simulink model "ADAC_AEBS_Test_B5_cs"  (R2014b)
settings: Solver=ode5  SolverMode=SingleTasking  StartTime=0.0  StopTime=inf  FixedStep=1/100  RelTol=1e-3
PreLoadFcn:
  | mbxruntime.callbacks.PreLoadFcn(bdroot);
  | check_NUTS_defined;
  | 
  | assignin('base',['model_closed_' bdroot],false);addpath('../includes_AEBS');
PostLoadFcn:
  | mbxruntime.callbacks.PostLoadFcn(bdroot);
InitFcn:
  | mbxruntime.callbacks.InitFcn(bdroot);
StartFcn:
  | mbxruntime.callbacks.StartFcn(bdroot);
StopFcn:
  | mbxruntime.callbacks.StopFcn(bdroot);
model workspace: external: MAT-File .\ADAC_AEBS_Test_B5_cs_hws.mat (data not in the file)
undefined symbols (not defined in the file or in its folder): OrientationPitch, OrientationRoll, PositionX, PositionY, PositionZ, warningInitialVelocity, x0
undefined symbols (not defined in the file): ADAC_AEBS_Test_B5_cs_1f353852a1e4a3c9, ADAC_AEBS_Test_B5_cs_31880a8290cb7cd0, ADAC_AEBS_Test_B5_cs_5496c81c4b1e331d, ADAC_AEBS_Test_B5_cs_a5262f062dfd1c06, ADAC_AEBS_Test_B5_cs_abe98bde40d8f1df, ADAC_AEBS_Test_B5_cs_ADAC_target_1_Path_pathUniqueID, ADAC_AEBS_Test_B5_cs_Audi_A8_1_Dynamics_Simple_initialPitch, ADAC_AEBS_Test_B5_cs_Audi_A8_1_Dynamics_Simple_initialRoll, ADAC_AEBS_Test_B5_cs_Audi_A8_1_Dynamics_Simple_initialX, ADAC_AEBS_Test_B5_cs_Audi_A8_1_Dynamics_Simple_initialY, ADAC_AEBS_Test_B5_cs_Audi_A8_1_Dynamics_Simple_initialYaw, ADAC_AEBS_Test_B5_cs_Audi_A8_1_Dynamics_Simple_initialZ, ADAC_AEBS_Test_B5_cs_Sphere_1_Dynamics_Empty_STATE_Sphere_1_x0, ADAC_AEBS_Test_B5_cs_Sphere_1_Dynamics_Empty_STATE_Sphere_1_y0, ADAC_AEBS_Test_B5_cs_Sphere_1_Dynamics_Empty_STATE_Sphere_1_z0, SteeringColumn, SteeringWheel, WheelL0, WheelL1, WheelR0, WheelR1
libraries: simulink x20, simulink_extras x12, PreScanSimulinkLibrary x5, PreScanUsefulBlocks x2
(part 4 of 6)

== system ADAC_AEBS_Test_B5_cs/Sphere_1/Dynamics_Empty ==
  note: For state mode 'Dynamic' positions
      | are not taken into account, as they
      | are computed by integrating velocity.
      | Click annotation for Help.
  " " : Constant  Value=0
  Add : Sum
  Add1 : Sum
  Bus Selector : BusSelector  OutputSignals=PositionX,PositionY
  Bus Assignment : BusAssignment  AssignedSignals=PositionX,PositionY,PositionZ,OrientationRoll,OrientationPitch
  MuxState : Subsystem  Tag=mux/State  Commented=on  mask(Empty Dynamics State Block){positioningmode=on, TimeStep=1/100}
      mask prompts: positioningmode "Positioning Mode"; TimeStep "Auto Assigned: Time Step [s]"
      mask help:
      | Build the state of an actor based on user input.
      | The user can either use positioning mode or dynamics mode.
      | - When using positioning mode the position and orientation of the actor are set directly based on the input. Expected input is relative to the initial position and orientation of the actor. It's also possible to specify the velocity of the actor, though this input isn't used, only passed on.
      | - When using dynamics mode the position input is ignored. Expected input is velocity and orientation. The velocity is relative the current orientation of the actor, while orientation is relative to its initial orientation. The position of the actor is calculated based on the velocity and orientation given.
      settings: DeleteFcn=PreScanBlockDeleteFcn;
  OffsetX : Constant  Value=0
  OffsetY : Constant  Value=0
  STATE_Sphere_1 : Subsystem  Tag=mux/StatePort  Priority=0  Commented=on  LoadFcn=load PrescanStateActuatorData  mask(PreScan Sink Block: State){x0=ADAC_AEBS_Test_B5_cs_Sphere_1_Dynamics_Empty_STATE_Sphere_1_x0, y0=ADAC_AEBS_Test_B5_cs_Sphere_1_Dynamics_Empty_STATE_Sphere_1_y0, z0=ADAC_AEBS_Test_B5_cs_Sphere_1_Dynamics_Empty_STATE_Sphere_1_z0, Roll0=ADAC_AEBS_Test_B5_cs_1f353852a1e4a3c9, Pitch0=ADAC_AEBS_Test_B5_cs_5496c81c4b1e331d, Yaw0=ADAC_AEBS_Test_B5_cs_31880a8290cb7cd0, TimeStep=1/100}
      mask prompts: x0 "Ini x-position VEHICLE wrt GLOBAL axis system [m]"; y0 "Ini y-position VEHICLE wrt GLOBAL axis system [m]"; z0 "Ini z-position VEHICLE wrt GLOBAL axis system [m]"; Roll0 "Ini roll-angle BODY wrt VEHICLE axis system [deg]"; Pitch0 "Ini pitch-angle BODY wrt VEHICLE axis system [deg]"; Yaw0 "Ini yaw-angle VEHICLE wrt GLOBAL axis system [deg]"; TimeStep "Auto-Assigned: Upload Period [s]"
      mask help:
      | The Actor State contains a vector signal of size (9x1), containing the following signals:
      |
      | -  Position                  (x,y,z)                                     [m]
      | -  Velocity                  (vx,vy,vz)                               [m/s]
      | -  Angles                    (Roll, Pitch, Yaw)                   [rad]
      |
      | The Actor state is defined in the global axis system.
      | The state is superponed on the Initial position defined in the GUI.
      |
      | For more information, please click Help.
      settings: DeleteFcn=PreScanBlockDeleteFcn;
      mask Help: eval('openHelp(222)')
      mask Display: image(imread('State.png'))
  State : Outport  Tag=outport/StateOutport  SampleTime=1/100
  wires:
  " "/1 -> Bus Assignment/4, Bus Assignment/5, Bus Assignment/6
  [view] -> Bus Assignment/1, Bus Selector/1
  Bus Selector/1 -> Add/1
  Add/1 -> Bus Assignment/2
  OffsetX/1 -> Add/2
  Bus Selector/2 -> Add1/1
  Add1/1 -> Bus Assignment/3
  OffsetY/1 -> Add1/2
  Bus Assignment/1 -> State/1
  MuxState/1(state) -> STATE_Sphere_1/1(State)

== system ADAC_AEBS_Test_B5_cs/Sphere_1/SELF_Demux ==
  SELF : Inport  OutDataTypeStr=Bus: PRESCAN_SELFSENSORDATA
  Bus Selector : BusSelector  OutputSignals=PositionX,PositionY,PositionZ,OrientationRoll,OrientationPitch,OrientationYaw,Velocity,Yaw_rate,Lat,Long,Alt
  Demux2 : Demux  Outputs=3
  Gain : Gain  Gain=180/pi
  Gain1 : Gain  Gain=180/pi
  Vector Concatenate1 : Concatenate  NumInputs=3
  compas converter : Subsystem
  x [m] : Outport
  y [m] : Outport  Port=2
  z [m] : Outport  Port=3
  rotx [deg] : Outport  Port=4
  roty [deg] : Outport  Port=5
  rotz [deg] : Outport  Port=6
  GPS lat [deg] : Outport  Port=7
  GPS long [deg] : Outport  Port=8
  GPS alt [m] : Outport  Port=9
  velocity [m/s] : Outport  Port=10
  heading [deg] : Outport  Port=11
  yaw rate [deg/s] : Outport  Port=12
  wires:
  Bus Selector/11 -> GPS alt [m]/1  "<Alt>"
  Bus Selector/10 -> GPS long [deg]/1  "<Long>"
  Bus Selector/9 -> GPS lat [deg]/1  "<Lat>"
  Bus Selector/8 -> Gain1/1  "<Yaw_rate>"
  Bus Selector/7 -> velocity [m/s]/1  "<Velocity>"
  Bus Selector/6 -> compas converter/1(rotz [rad]), Vector Concatenate1/3  "<OrientationYaw>"
  Bus Selector/5 -> Vector Concatenate1/2  "<OrientationPitch>"
  Bus Selector/4 -> Vector Concatenate1/1  "<OrientationRoll>"
  Vector Concatenate1/1 -> Gain/1
  Bus Selector/3 -> z [m]/1  "<PositionZ>"
  Bus Selector/2 -> y [m]/1  "<PositionY>"
  Bus Selector/1 -> x [m]/1  "<PositionX>"
  SELF/1 -> Bus Selector/1
  Gain/1 -> Demux2/1
  Demux2/1 -> rotx [deg]/1
  Demux2/2 -> roty [deg]/1
  Demux2/3 -> rotz [deg]/1
  compas converter/1(heading [deg]) -> heading [deg]/1
  Gain1/1 -> yaw rate [deg/s]/1

== system ADAC_AEBS_Test_B5_cs/SteeringColumn_pivot_Audi_A8_1/Actuator ==
  Joint : Inport
  Bus Selector : BusSelector  OutputSignals=POSITION,ORIENTATION
  visu_Rotate : Subsystem  mask(RPYActuator){UniqueID=UniqueID, Object3DID=Rotate_ObjectID3D, TimeStep=TimeStep}
      mask prompts: UniqueID "Auto-Assigned: Unique ID"; Object3DID "Auto-Assigned: Child 3D Object ID"; TimeStep "Auto-Assigned: Upload Period [s]"
      mask help: Applies angles update to selected child object
      mask Help:
      | Applies position update to selected child object
      | 
      | - UniqueID (double)   : Unique ID of the parent actor
      | - Object3DID (string) : Name of the child 3D object
      mask Display: port_label('input', 1, ['visu_Rotate_' Object3DID])
  visu_Translate : Subsystem  mask(PositionActuator){UniqueID=UniqueID, Object3DID=Translate_ObjectID3D, TimeStep=TimeStep}
      mask prompts: UniqueID "Auto-Assigned: Unique ID"; Object3DID "Auto-Assigned: Child 3D Object ID"; TimeStep "Auto-Assigned: Upload Period [s]"
      mask help: Applies position update to selected child object
      mask Help:
      | Applies position update to selected child object
      | 
      | - UniqueID (double)   : Unique ID of the parent actor
      | - Object3DID (string) : Name of the child 3D object
      mask Display: port_label('input', 1, ['visu_Translate_' Object3DID])
  wires:
  Bus Selector/2 -> visu_Rotate/1(In1)  "<ORIENTATION>"
  Bus Selector/1 -> visu_Translate/1(In1)  "<POSITION>"
  Joint/1 -> Bus Selector/1

== system ADAC_AEBS_Test_B5_cs/SteeringWheel_pivot_Audi_A8_1/Actuator ==
  Joint : Inport
  Bus Selector : BusSelector  OutputSignals=POSITION,ORIENTATION
  visu_Rotate : Subsystem  mask(RPYActuator){UniqueID=UniqueID, Object3DID=Rotate_ObjectID3D, TimeStep=TimeStep}
      mask prompts: UniqueID "Auto-Assigned: Unique ID"; Object3DID "Auto-Assigned: Child 3D Object ID"; TimeStep "Auto-Assigned: Upload Period [s]"
      mask help: Applies angles update to selected child object
      mask Help:
      | Applies position update to selected child object
      | 
      | - UniqueID (double)   : Unique ID of the parent actor
      | - Object3DID (string) : Name of the child 3D object
      mask Display: port_label('input', 1, ['visu_Rotate_' Object3DID])
  visu_Translate : Subsystem  mask(PositionActuator){UniqueID=UniqueID, Object3DID=Translate_ObjectID3D, TimeStep=TimeStep}
      mask prompts: UniqueID "Auto-Assigned: Unique ID"; Object3DID "Auto-Assigned: Child 3D Object ID"; TimeStep "Auto-Assigned: Upload Period [s]"
      mask help: Applies position update to selected child object
      mask Help:
      | Applies position update to selected child object
      | 
      | - UniqueID (double)   : Unique ID of the parent actor
      | - Object3DID (string) : Name of the child 3D object
      mask Display: port_label('input', 1, ['visu_Translate_' Object3DID])
  wires:
  Bus Selector/2 -> visu_Rotate/1(In1)  "<ORIENTATION>"
  Bus Selector/1 -> visu_Translate/1(In1)  "<POSITION>"
  Joint/1 -> Bus Selector/1

== system ADAC_AEBS_Test_B5_cs/WheelL0_Audi_A8_1/Actuator ==
  Joint : Inport
  Bus Selector : BusSelector  OutputSignals=POSITION,ORIENTATION
  visu_Rotate : Subsystem  mask(RPYActuator){UniqueID=UniqueID, Object3DID=Rotate_ObjectID3D, TimeStep=TimeStep}
      mask prompts: UniqueID "Auto-Assigned: Unique ID"; Object3DID "Auto-Assigned: Child 3D Object ID"; TimeStep "Auto-Assigned: Upload Period [s]"
      mask help: Applies angles update to selected child object
      mask Help:
      | Applies position update to selected child object
      | 
      | - UniqueID (double)   : Unique ID of the parent actor
      | - Object3DID (string) : Name of the child 3D object
      mask Display: port_label('input', 1, ['visu_Rotate_' Object3DID])
  visu_Translate : Subsystem  mask(PositionActuator){UniqueID=UniqueID, Object3DID=Translate_ObjectID3D, TimeStep=TimeStep}
      mask prompts: UniqueID "Auto-Assigned: Unique ID"; Object3DID "Auto-Assigned: Child 3D Object ID"; TimeStep "Auto-Assigned: Upload Period [s]"
      mask help: Applies position update to selected child object
      mask Help:
      | Applies position update to selected child object
      | 
      | - UniqueID (double)   : Unique ID of the parent actor
      | - Object3DID (string) : Name of the child 3D object
      mask Display: port_label('input', 1, ['visu_Translate_' Object3DID])
  wires:
  Bus Selector/2 -> visu_Rotate/1(In1)  "<ORIENTATION>"
  Bus Selector/1 -> visu_Translate/1(In1)  "<POSITION>"
  Joint/1 -> Bus Selector/1

== system ADAC_AEBS_Test_B5_cs/WheelL1_Audi_A8_1/Actuator ==
  Joint : Inport
  Bus Selector : BusSelector  OutputSignals=POSITION,ORIENTATION
  visu_Rotate : Subsystem  mask(RPYActuator){UniqueID=UniqueID, Object3DID=Rotate_ObjectID3D, TimeStep=TimeStep}
      mask prompts: UniqueID "Auto-Assigned: Unique ID"; Object3DID "Auto-Assigned: Child 3D Object ID"; TimeStep "Auto-Assigned: Upload Period [s]"
      mask help: Applies angles update to selected child object
      mask Help:
      | Applies position update to selected child object
      | 
      | - UniqueID (double)   : Unique ID of the parent actor
      | - Object3DID (string) : Name of the child 3D object
      mask Display: port_label('input', 1, ['visu_Rotate_' Object3DID])
  visu_Translate : Subsystem  mask(PositionActuator){UniqueID=UniqueID, Object3DID=Translate_ObjectID3D, TimeStep=TimeStep}
      mask prompts: UniqueID "Auto-Assigned: Unique ID"; Object3DID "Auto-Assigned: Child 3D Object ID"; TimeStep "Auto-Assigned: Upload Period [s]"
      mask help: Applies position update to selected child object
      mask Help:
      | Applies position update to selected child object
      | 
      | - UniqueID (double)   : Unique ID of the parent actor
      | - Object3DID (string) : Name of the child 3D object
      mask Display: port_label('input', 1, ['visu_Translate_' Object3DID])
  wires:
  Bus Selector/2 -> visu_Rotate/1(In1)  "<ORIENTATION>"
  Bus Selector/1 -> visu_Translate/1(In1)  "<POSITION>"
  Joint/1 -> Bus Selector/1

== system ADAC_AEBS_Test_B5_cs/WheelR0_Audi_A8_1/Actuator ==
  Joint : Inport
  Bus Selector : BusSelector  OutputSignals=POSITION,ORIENTATION
  visu_Rotate : Subsystem  mask(RPYActuator){UniqueID=UniqueID, Object3DID=Rotate_ObjectID3D, TimeStep=TimeStep}
      mask prompts: UniqueID "Auto-Assigned: Unique ID"; Object3DID "Auto-Assigned: Child 3D Object ID"; TimeStep "Auto-Assigned: Upload Period [s]"
      mask help: Applies angles update to selected child object
      mask Help:
      | Applies position update to selected child object
      | 
      | - UniqueID (double)   : Unique ID of the parent actor
      | - Object3DID (string) : Name of the child 3D object
      mask Display: port_label('input', 1, ['visu_Rotate_' Object3DID])
  visu_Translate : Subsystem  mask(PositionActuator){UniqueID=UniqueID, Object3DID=Translate_ObjectID3D, TimeStep=TimeStep}
      mask prompts: UniqueID "Auto-Assigned: Unique ID"; Object3DID "Auto-Assigned: Child 3D Object ID"; TimeStep "Auto-Assigned: Upload Period [s]"
      mask help: Applies position update to selected child object
      mask Help:
      | Applies position update to selected child object
      | 
      | - UniqueID (double)   : Unique ID of the parent actor
      | - Object3DID (string) : Name of the child 3D object
      mask Display: port_label('input', 1, ['visu_Translate_' Object3DID])
  wires:
  Bus Selector/2 -> visu_Rotate/1(In1)  "<ORIENTATION>"
  Bus Selector/1 -> visu_Translate/1(In1)  "<POSITION>"
  Joint/1 -> Bus Selector/1

== system ADAC_AEBS_Test_B5_cs/WheelR1_Audi_A8_1/Actuator ==
  Joint : Inport
  Bus Selector : BusSelector  OutputSignals=POSITION,ORIENTATION
  visu_Rotate : Subsystem  mask(RPYActuator){UniqueID=UniqueID, Object3DID=Rotate_ObjectID3D, TimeStep=TimeStep}
      mask prompts: UniqueID "Auto-Assigned: Unique ID"; Object3DID "Auto-Assigned: Child 3D Object ID"; TimeStep "Auto-Assigned: Upload Period [s]"
      mask help: Applies angles update to selected child object
      mask Help:
      | Applies position update to selected child object
      | 
      | - UniqueID (double)   : Unique ID of the parent actor
      | - Object3DID (string) : Name of the child 3D object
      mask Display: port_label('input', 1, ['visu_Rotate_' Object3DID])
  visu_Translate : Subsystem  mask(PositionActuator){UniqueID=UniqueID, Object3DID=Translate_ObjectID3D, TimeStep=TimeStep}
      mask prompts: UniqueID "Auto-Assigned: Unique ID"; Object3DID "Auto-Assigned: Child 3D Object ID"; TimeStep "Auto-Assigned: Upload Period [s]"
      mask help: Applies position update to selected child object
      mask Help:
      | Applies position update to selected child object
      | 
      | - UniqueID (double)   : Unique ID of the parent actor
      | - Object3DID (string) : Name of the child 3D object
      mask Display: port_label('input', 1, ['visu_Translate_' Object3DID])
  wires:
  Bus Selector/2 -> visu_Rotate/1(In1)  "<ORIENTATION>"
  Bus Selector/1 -> visu_Translate/1(In1)  "<POSITION>"
  Joint/1 -> Bus Selector/1

== system ADAC_AEBS_Test_B5_cs/ADAC_target_1/SELF_Demux/compas converter ==
  rotz [rad] : Inport
  cart2compas : Subsystem
  rad2deg : Gain  Gain=180/pi
  heading [deg] : Outport
  wires:
  rad2deg/1 -> cart2compas/1(Angle [deg])
  rotz [rad]/1 -> rad2deg/1
  cart2compas/1(heading [deg]) -> heading [deg]/1

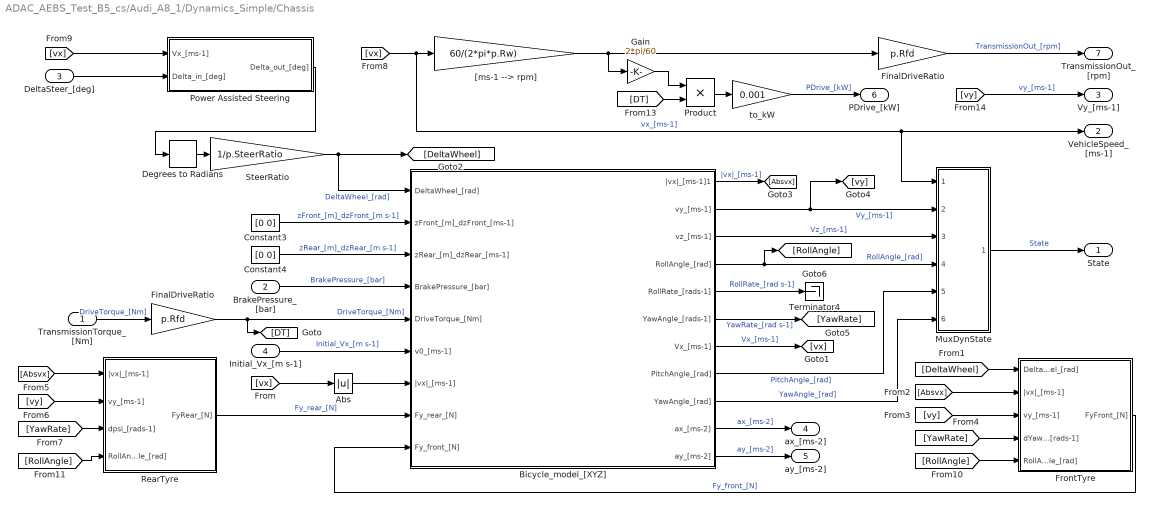
== system ADAC_AEBS_Test_B5_cs/Audi_A8_1/Dynamics_Simple/Chassis ==
  TransmissionTorque_[Nm] : Inport
  BrakePressure_[bar] : Inport  Port=2
  DeltaSteer_[deg] : Inport  Port=3
  Initial_Vx_[m s-1] : Inport  Port=4
  Abs : Abs
  Bicycle_model_[XYZ] : Subsystem
      mask Display: image(imread('Bicycle_model.png'));
  Constant3 : Constant  Value=[0 0]
  Constant4 : Constant  Value=[0 0]
  Degrees to Radians : simulink_extras/Transformations/Degrees to Radians
  FinalDriveRatio : Gain  Gain=p.Rfd  SaturateOnIntegerOverflow=on  OutDataTypeStr=Inherit: Same as input  ParamDataTypeStr=Inherit: Same as input
  "FinalDriveRatio " : Gain  Gain=p.Rfd  SaturateOnIntegerOverflow=on  OutDataTypeStr=Inherit: Same as input  ParamDataTypeStr=Inherit: Same as input
  FrontTyre : Subsystem
      mask Display: image(imread('Tyre.png'));
  Gain : Gain  Gain=2*pi/60
  MuxDynState : Subsystem
  Power Assisted Steering : Subsystem
  Product : Product  RndMeth=Zero
  RearTyre : Subsystem
      mask Display: image(imread('Tyre.png'));
  SteerRatio : Gain  Gain=1/p.SteerRatio
  Terminator4 : Terminator
  "[ms-1 --> rpm]" : Gain  Gain=60/(2*pi*p.Rw)  SaturateOnIntegerOverflow=on  OutDataTypeStr=Inherit: Same as input  ParamDataTypeStr=Inherit: Same as input
  to_kW : Gain  Gain=0.001
  State : Outport
  VehicleSpeed_[ms-1] : Outport  Port=2
  Vy_[ms-1] : Outport  Port=3
  ax_[ms-2] : Outport  Port=4
  ay_[ms-2] : Outport  Port=5
  PDrive_[kW] : Outport  Port=6
  TransmissionOut_[rpm] : Outport  Port=7
  wires:
  [vy] -> Vy_[ms-1]/1  "vy_[ms-1]"
  to_kW/1 -> PDrive_[kW]/1  "PDrive_[kW]"
  Gain/1 -> Product/1
  Bicycle_model_[XYZ]/10(ax_[ms-2]) -> ax_[ms-2]/1  "ax_[ms-2]"
  Product/1 -> to_kW/1
  [DT] -> Product/2
  Bicycle_model_[XYZ]/11(ay_[ms-2]) -> ay_[ms-2]/1  "ay_[ms-2]"
  Abs/1 -> Bicycle_model_[XYZ]/7(|vx|_[ms-1])
  Degrees to Radians/1 -> SteerRatio/1
  [vx] -> Abs/1
  SteerRatio/1 -> [DeltaWheel], Bicycle_model_[XYZ]/1(DeltaWheel_[rad])  "DeltaWheel_[rad]"
  TransmissionTorque_[Nm]/1 -> "FinalDriveRatio "/1  "DriveTorque_[Nm]"
  RearTyre/1(FyRear_[N]) -> Bicycle_model_[XYZ]/8(Fy_rear_[N])  "Fy_rear_[N]"
  FrontTyre/1(FyFront_[N]) -> Bicycle_model_[XYZ]/9(Fy_front_[N])  "Fy_front_[N]"
  Bicycle_model_[XYZ]/1(|vx|_[ms-1]1) -> [Absvx]  "|vx|_[ms-1]"
  Bicycle_model_[XYZ]/2(vy_[ms-1]) -> [vy], MuxDynState/2(vy [ms-1])  "Vy_[ms-1]"
  Bicycle_model_[XYZ]/4(RollAngle_[rad]) -> MuxDynState/4(R [rad]), [RollAngle]  "RollAngle_[rad]"
  Bicycle_model_[XYZ]/6(YawAngle_[rads-1]) -> [YawRate]  "YawRate_[rad s-1]"
  Bicycle_model_[XYZ]/7(Vx_[ms-1]) -> [vx]  "Vx_[ms-1]"
  [DeltaWheel] -> FrontTyre/1(DeltaWheel_[rad])
  [Absvx] -> FrontTyre/2(|vx|_[ms-1])
  [vy] -> FrontTyre/3(vy_[ms-1])
  [YawRate] -> FrontTyre/4(dYawAngle_[rads-1])
  [Absvx] -> RearTyre/1(|vx|_[ms-1])
  [vy] -> RearTyre/2(vy_[ms-1])
  [YawRate] -> RearTyre/3(dpsi_[rads-1])
  Bicycle_model_[XYZ]/3(vz_[ms-1]) -> MuxDynState/3(vz [ms-1])  "Vz_[ms-1]"
  Bicycle_model_[XYZ]/8(PitchAngle_[rad]) -> MuxDynState/5(P [rad])  "PitchAngle_[rad]"
  Bicycle_model_[XYZ]/9(YawAngle_[rad]) -> MuxDynState/6(Y [rad])  "YawAngle_[rad]"
  "[ms-1 --> rpm]"/1 -> Gain/1, FinalDriveRatio/1
  FinalDriveRatio/1 -> TransmissionOut_[rpm]/1  "TransmissionOut_[rpm]"
  [vx] -> "[ms-1 --> rpm]"/1, VehicleSpeed_[ms-1]/1, MuxDynState/1(vx [ms-1])  "vx_[ms-1]"
  [vx] -> Power Assisted Steering/1(Vx_[ms-1])
  DeltaSteer_[deg]/1 -> Power Assisted Steering/2(Delta_in_[deg])
  Power Assisted Steering/1(Delta_out_[deg]) -> Degrees to Radians/1
  [RollAngle] -> FrontTyre/5(RollAngle_[rad])
  [RollAngle] -> RearTyre/4(RollAngle_[rad])
  Constant3/1 -> Bicycle_model_[XYZ]/2(zFront_[m]_dzFront_[ms-1])  "zFront_[m]_dzFront_[m s-1]"
  Constant4/1 -> Bicycle_model_[XYZ]/3(zRear_[m]_dzRear_[ms-1])  "zRear_[m]_dzRear_[m s-1]"
  BrakePressure_[bar]/1 -> Bicycle_model_[XYZ]/4(BrakePressure_[bar])  "BrakePressure_[bar]"
  "FinalDriveRatio "/1 -> Bicycle_model_[XYZ]/5(DriveTorque_[Nm]), [DT]  "DriveTorque_[Nm]"
  Initial_Vx_[m s-1]/1 -> Bicycle_model_[XYZ]/6(v0_[ms-1])  "Initial_Vx_[m s-1]"
  Bicycle_model_[XYZ]/5(RollRate_[rads-1]) -> Terminator4/1  "RollRate_[rad s-1]"
  MuxDynState/1(State) -> State/1  "State"

== system ADAC_AEBS_Test_B5_cs/Audi_A8_1/Dynamics_Simple/Engine ==
  ImpellerTorque_[Nm] : Inport
  Throttle_[%] : Inport  Port=2
  Configurable Subsystem : Subsystem  BlockChoice=Discrete Rate Limiter  mask{ComputationMode=ComputationMode}
      mask prompts: ComputationMode "Compuation mode:"
      mask init:
      | SetComputationMode(gcb,ComputationMode);
      settings: AttributesFormatString=%<BlockChoice>  OpenFcn=BringToFront(gcb);  MemberBlocks=Discrete Rate Limiter,Rate Limiter
      settings: TemplateBlock=|
      | PreScanSimulinkLibrary/Configurable Subsystems/TransferFunction
      | Engine/Configurable
      | Subsystem
  Configurable Subsystem1 : Subsystem  BlockChoice=Discrete-Time Integrator  mask{ComputationMode=ComputationMode}
      mask prompts: ComputationMode "Computation mode:"
      mask init:
      | SetComputationMode(gcb,ComputationMode);
      settings: AttributesFormatString=%<BlockChoice>  OpenFcn=BringToFront(gcb);  MemberBlocks=Discrete-Time Integrator,Integrator
      settings: TemplateBlock=|
      | PreScanSimulinkLibrary/Configurable Subsystems/integral with initial condition and limts
      | for engine/Configurable
      | Subsystem
  EngineTorque : Lookup2D  RowIndex=p.thvec  ColumnIndex=p.nevec  Table=p.emap  InputSameDT=on
  Gain : Gain  Gain=2*pi/60
  Product : Product  RndMeth=Zero
  Sum : Sum  Inputs=-+  SaturateOnIntegerOverflow=on  InputSameDT=on  OutDataTypeStr=Inherit: Same as first input
  engine + impeller inertia : Gain  Gain=1/p.Iei  SaturateOnIntegerOverflow=on  OutDataTypeStr=Inherit: Same as input  ParamDataTypeStr=Inherit: Same as input
  rad|sec2rpm : Gain  Gain=60/2/pi  SaturateOnIntegerOverflow=on  OutDataTypeStr=Inherit: Same as input  ParamDataTypeStr=Inherit: Same as input
  to_kW : Gain  Gain=0.001
  nEngine_[rpm] : Outport  InitialOutput=0
  PEngine_[kW] : Outport  Port=2  InitialOutput=0
  wires:
  rad|sec2rpm/1 -> nEngine_[rpm]/1, EngineTorque/2, Gain/1  "rpm"
  engine + impeller inertia/1 -> Configurable Subsystem1/1(In1)  "rads-2"
  EngineTorque/1 -> Sum/2, Product/2
  Sum/1 -> engine + impeller inertia/1
  Configurable Subsystem1/1(Out1) -> rad|sec2rpm/1  "rads-1"
  Throttle_[%]/1 -> Configurable Subsystem/1(In1)
  ImpellerTorque_[Nm]/1 -> Sum/1
  Configurable Subsystem/1(Out1) -> EngineTorque/1
  Product/1 -> to_kW/1
  Gain/1 -> Product/1
  to_kW/1 -> PEngine_[kW]/1

== system ADAC_AEBS_Test_B5_cs/Audi_A8_1/Dynamics_Simple/Gear: Auto Manual ==
  note: 0; Auto = on // Manual =off
      | 1; Auto = off // Manual =on
  Auto_Manual : Inport
  Manual_Gear : Inport  Port=2
  Auto_Gear : Inport  Port=3
  If : If  IfExpression=u1 == 0
  If Action Subsystem : Subsystem  TreatAsAtomicUnit=on
  If Action Subsystem1 : Subsystem  TreatAsAtomicUnit=on
  Merge : Merge
  Gear : Outport
  wires:
  If Action Subsystem/1(Out1) -> Merge/1
  Auto_Gear/1 -> If Action Subsystem/1(In1)
  If/1 -> If Action Subsystem/Action
  Merge/1 -> Gear/1
  If Action Subsystem1/1(Out1) -> Merge/2
  Manual_Gear/1 -> If Action Subsystem1/1(In1)
  If/2 -> If Action Subsystem1/Action
  Auto_Manual/1 -> If/1

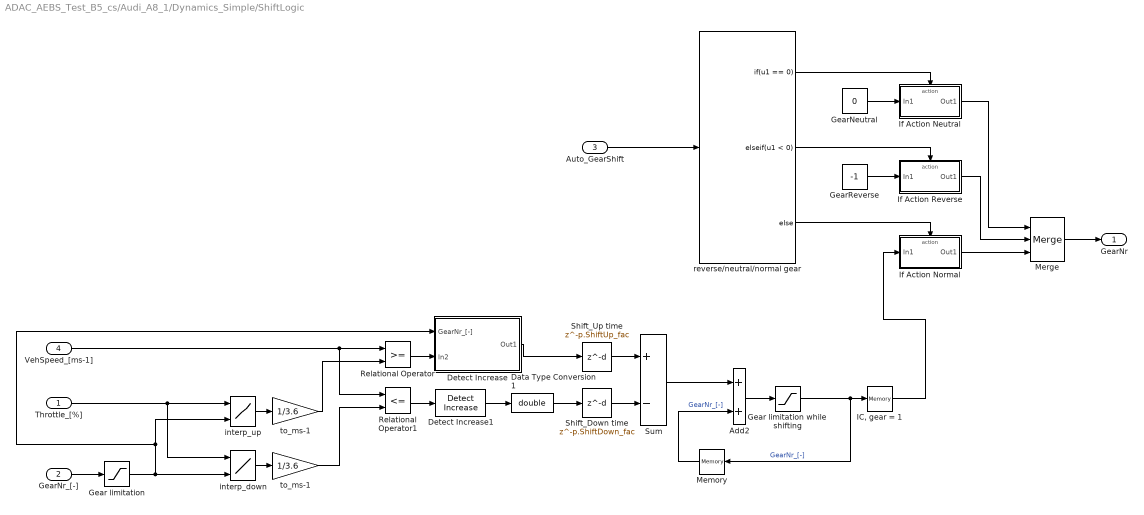
== system ADAC_AEBS_Test_B5_cs/Audi_A8_1/Dynamics_Simple/ShiftLogic ==
  Throttle_[%] : Inport
  GearNr_[-] : Inport  Port=2
  Auto_GearShift : Inport  Port=3
  VehSpeed_[ms-1] : Inport  Port=4
  Add2 : Sum
  Data Type Conversion1 : DataTypeConversion  OutDataTypeStr=double
  Detect Increase1 : simulink/Logic and Bit Operations/Detect Increase  vinit=0.0  InputProcessing=Inherited  OutDataTypeStr=uint8
  Detect Increase : Subsystem
  Gear limitation : Saturate  UpperLimit=p.maxGear  LowerLimit=1
  Gear limitation while shifting : Saturate  UpperLimit=p.maxGear  LowerLimit=1
  GearNeutral : Constant  Value=0
  GearReverse : Constant  Value=-1
  "IC, gear = 1" : Memory  X0=1  InheritSampleTime=on
  If Action Neutral : Subsystem  TreatAsAtomicUnit=on
  If Action Normal : Subsystem  TreatAsAtomicUnit=on
  If Action Reverse : Subsystem  TreatAsAtomicUnit=on
  Memory : Memory  InheritSampleTime=on
  Merge : Merge  Inputs=3
  Relational Operator : RelationalOperator  OutDataTypeStr=boolean
  Relational Operator1 : RelationalOperator  Operator=<=  OutDataTypeStr=boolean
  Shift_Down time : Delay  DelayLength=p.ShiftDown_fac  InputProcessing=Inherited
  Shift_Up time : Delay  DelayLength=p.ShiftUp_fac  InputProcessing=Inherited
  Sum : Sum  Inputs=+-
  interp_down : Lookup2D  RowIndex=p.downth  ColumnIndex=[1:p.maxGear]  Table=p.downtab  LookUpMeth=Interpolation-Use End Values  InputSameDT=on
  interp_up : Lookup2D  RowIndex=p.upth  ColumnIndex=[1:p.maxGear]  Table=p.uptab  LookUpMeth=Interpolation-Use End Values  InputSameDT=on
  reverse/neutral/normal gear : If  IfExpression=u1 == 0  ElseIfExpressions=u1 < 0
  to_ms-1 : Gain  Gain=1/3.6
  "to_ms-1 " : Gain  Gain=1/3.6
  GearNr : Outport
  wires:
  Auto_GearShift/1 -> reverse/neutral/normal gear/1
  "IC, gear = 1"/1 -> If Action Normal/1(In1)
  Merge/1 -> GearNr/1
  If Action Reverse/1(Out1) -> Merge/2
  If Action Neutral/1(Out1) -> Merge/1
  If Action Normal/1(Out1) -> Merge/3
  reverse/neutral/normal gear/3 -> If Action Normal/Action
  reverse/neutral/normal gear/1 -> If Action Neutral/Action
  reverse/neutral/normal gear/2 -> If Action Reverse/Action
  GearReverse/1 -> If Action Reverse/1(In1)
  GearNeutral/1 -> If Action Neutral/1(In1)
  Shift_Down time/1 -> Sum/2
  Shift_Up time/1 -> Sum/1
  Detect Increase/1(Out1) -> Shift_Up time/1
  Data Type Conversion1/1 -> Shift_Down time/1
  Detect Increase1/1 -> Data Type Conversion1/1
  Sum/1 -> Add2/1
  Memory/1 -> Add2/2  "GearNr_[-]"
  Add2/1 -> Gear limitation while shifting/1
  Gear limitation while shifting/1 -> "IC, gear = 1"/1, Memory/1  "GearNr_[-]"
  Throttle_[%]/1 -> interp_down/1, interp_up/1
  Relational Operator/1 -> Detect Increase/2(In2)
  Relational Operator1/1 -> Detect Increase1/1
  interp_down/1 -> "to_ms-1 "/1
  VehSpeed_[ms-1]/1 -> Relational Operator/1, Relational Operator1/1
  interp_up/1 -> to_ms-1/1
  Gear limitation/1 -> interp_down/2, interp_up/2, Detect Increase/1(GearNr_[-])
  GearNr_[-]/1 -> Gear limitation/1
  to_ms-1/1 -> Relational Operator/2
  "to_ms-1 "/1 -> Relational Operator1/2

== system ADAC_AEBS_Test_B5_cs/Audi_A8_1/Dynamics_Simple/Transmission ==
  nEngine_[rpm] : Inport
  GearNr_[-] : Inport  Port=2
  n_TransmissionOut_[rpm] : Inport  Port=3
  Torque_Converter : Subsystem
      mask Display: image(imread('TorqueConverter.png'));
  Transmission_Ratio : Subsystem
  Viscous coupling : Lookup  InputValues=[-5:0.1:5]*p.m/4  Table=p.m/4*tanh([-5:0.1:5])
  ImpellerTorque_[Nm] : Outport  InitialOutput=0
  TransmissionTorque_[Nm] : Outport  Port=2  InitialOutput=0
  wires:
  Torque_Converter/2(TurbineTorque_[Nm]) -> Viscous coupling/1  "Converter_Torque_[Nm]"
  Transmission_Ratio/2(nTransmissionIn_[rpm]) -> Torque_Converter/2(nTransmission_[rpm])
  nEngine_[rpm]/1 -> Torque_Converter/1(nEngine_[rpm])
  GearNr_[-]/1 -> Transmission_Ratio/2(GearNr_[-]), Torque_Converter/3(Gear nr)
  n_TransmissionOut_[rpm]/1 -> Transmission_Ratio/3(nTransmissionOut_[rpm])
  Torque_Converter/1(ImpellerTorque_[Nm]) -> ImpellerTorque_[Nm]/1
  Transmission_Ratio/1(tTransmissionOut_[Nm]) -> TransmissionTorque_[Nm]/1
  Viscous coupling/1 -> Transmission_Ratio/1(tTransmissionIn_[Nm])

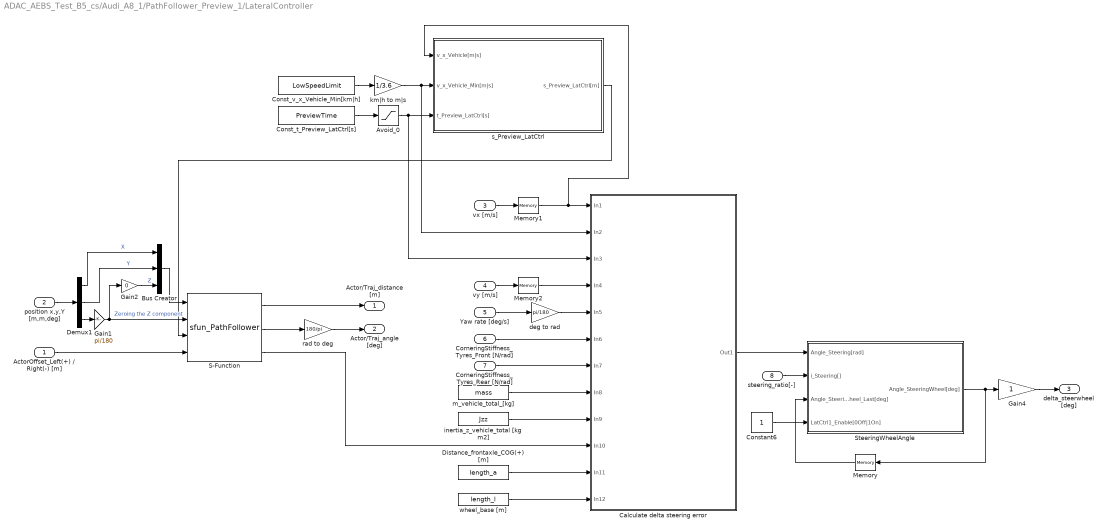
== system ADAC_AEBS_Test_B5_cs/Audi_A8_1/PathFollower_Preview_1/LateralController ==
  ActorOffset_Left(+) / Right(-) [m] : Inport
  position x,y,Y [m,m,deg] : Inport  Port=2
  vx [m/s] : Inport  Port=3
  vy [m/s] : Inport  Port=4
  Yaw rate [deg/s] : Inport  Port=5
  CorneringStiffness_Tyres_Front [N/rad] : Inport  Port=6
  CorneringStiffness_Tyres_Rear [N/rad] : Inport  Port=7
  steering_ratio[-] : Inport  Port=8
  Avoid_0 : Saturate  UpperLimit=1000  LowerLimit=0.1
  Bus Creator : BusCreator  Inputs='X','Y','Z'  OutDataTypeStr=Bus: PRESCAN_XYZ_DATA
  Calculate delta steering error : Subsystem
      mask Display:
      | port_label('input', 1, 'v_x_vehicle [m/s]')
      | port_label('input', 2, 'v_x_vehicle_Min [m/s]')
      | port_label('input', 3, 't_Preview_LatCtrl [s]')
      | port_label('input', 4, 'v_y_vehicle [m/s]')
      | port_label('input', 5, 'yawrate_vehicle [rad/sec]')
      | port_label('input', 6, 'CorneringStiffness_Tyres_Front [N/rad]')
      | port_label('input', 7, 'CorneringStiffness_Tyres_Rear [N/rad]')
      | port_label('input', 8, 'm_vehicle_total [kg]')
      | port_label('input', 9, 'inertia_z_vehicle_total [kg m2]')
      | port_label('input', 10, 'e_Lat [m]')
      | port_label('input', 11, 'Distance_frontaxle_COG(+) [m]')
      | port_label('input', 12, 'wheel_base [m]')
      | port_label('output', 1, 'delta_steeringwheel [rad]')
  Const_t_Preview_LatCtrl[s] : Constant  Value=PreviewTime  SampleTime=CSSampleTime
  Const_v_x_Vehicle_Min[km|h] : Constant  Value=LowSpeedLimit  SampleTime=CSSampleTime
  Constant6 : Constant  SampleTime=CSSampleTime
  Demux1 : Demux  Outputs=3
  Distance_frontaxle_COG(+) [m] : Constant  Value=length_a  SampleTime=CSSampleTime
  Gain1 : Gain  Gain=pi/180
  Gain2 : Gain  Gain=0
  Gain4 : Gain
  Memory : Memory  InheritSampleTime=on
  Memory1 : Memory  InheritSampleTime=on
  Memory2 : Memory  InheritSampleTime=on
  S-Function : S-Function  FunctionName=sfun_PathFollower  Parameters=PathUniqueID,-1  EnableBusSupport=off
  SteeringWheelAngle : Subsystem
  deg to rad : Gain  Gain=pi/180
  inertia_z_vehicle_total [kg m2] : Constant  Value=Jzz  SampleTime=CSSampleTime
  km|h to m|s : Gain  Gain=1/3.6
  m_vehicle_total_[kg] : Constant  Value=mass  SampleTime=CSSampleTime
  rad to deg : Gain  Gain=180/pi
  s_Preview_LatCtrl : Subsystem
  wheel_base [m] : Constant  Value=length_l  SampleTime=CSSampleTime
  Actor/Traj_distance [m] : Outport
  Actor/Traj_angle [deg] : Outport  Port=2
  delta_steerwheel [deg] : Outport  Port=3
  wires:
  Gain2/1 -> Bus Creator/3  "Z"
  Bus Creator/1 -> S-Function/1
  Demux1/2 -> Bus Creator/2  "Y"
  Demux1/1 -> Bus Creator/1  "X"
  s_Preview_LatCtrl/1(s_Preview_LatCtrl[m]) -> S-Function/3
  rad to deg/1 -> Actor/Traj_angle [deg]/1
  km|h to m|s/1 -> Calculate delta steering error/2(In2), s_Preview_LatCtrl/2(v_x_Vehicle_Min[m|s])
  ActorOffset_Left(+) / Right(-) [m]/1 -> S-Function/4
  S-Function/2 -> rad to deg/1
  S-Function/1 -> Actor/Traj_distance [m]/1
  Calculate delta steering error/1(Out1) -> SteeringWheelAngle/1(Angle_Steering[rad])
  vx [m/s]/1 -> Memory1/1
  vy [m/s]/1 -> Memory2/1
  CorneringStiffness_Tyres_Front [N/rad]/1 -> Calculate delta steering error/6(In6)
  m_vehicle_total_[kg]/1 -> Calculate delta steering error/8(In8)
  inertia_z_vehicle_total [kg m2]/1 -> Calculate delta steering error/9(In9)
  steering_ratio[-]/1 -> SteeringWheelAngle/2(i_Steering[])
  SteeringWheelAngle/1(Angle_SteeringWheel[deg]) -> Gain4/1, Memory/1
  Memory/1 -> SteeringWheelAngle/3(Angle_SteeringWheel_Last[deg])
  Constant6/1 -> SteeringWheelAngle/4(LatCtrl1_Enable[0Off|1On])
  Avoid_0/1 -> Calculate delta steering error/3(In3), s_Preview_LatCtrl/3(t_Preview_LatCtrl[s])
  Const_v_x_Vehicle_Min[km|h]/1 -> km|h to m|s/1
  Const_t_Preview_LatCtrl[s]/1 -> Avoid_0/1
  Gain4/1 -> delta_steerwheel [deg]/1
  Distance_frontaxle_COG(+) [m]/1 -> Calculate delta steering error/11(In11)
  CorneringStiffness_Tyres_Rear [N/rad]/1 -> Calculate delta steering error/7(In7)
  Yaw rate [deg/s]/1 -> deg to rad/1
  deg to rad/1 -> Calculate delta steering error/5(In5)
  Gain1/1 -> Gain2/1, S-Function/2  "Zeroing the Z component"
  Demux1/3 -> Gain1/1
  position x,y,Y [m,m,deg]/1 -> Demux1/1
  wheel_base [m]/1 -> Calculate delta steering error/12(In12)
  S-Function/3 -> Calculate delta steering error/10(In10)
  Memory1/1 -> Calculate delta steering error/1(In1), s_Preview_LatCtrl/1(v_x_Vehicle[m|s])
  Memory2/1 -> Calculate delta steering error/4(In4)

== system ADAC_AEBS_Test_B5_cs/Audi_A8_1/PathFollower_Preview_1/LongitudinalController ==
  v_actual [m/s] : Inport
  Desired Velocity [m/s] : Inport  Port=2
  Initial Velocity [m/s] : Inport  Port=3
  Check_Initial_Velocity : Subsystem
  Demux : Demux  Outputs=3
  GearNormal : Constant
  "GearNormal " : Constant
  If Desired Velocity = 0 : Subsystem  TreatAsAtomicUnit=on
  If Desired Velocity ~= 0 : Subsystem  TreatAsAtomicUnit=on
  Memory External IC : Subsystem
  Merge : Merge
  Mux : Mux  Inputs=3
  Mux2 : Mux  Inputs=3
  Sum4 : Sum  Inputs=|+-
  if : If  IfExpression=u1 == 0  SampleTime=CSSampleTime
  throttle [%] : Outport
  brake pressure [bar] : Outport  Port=2
  v0 [m/s] : Outport  Port=3
  Auto_GearShift : Outport  Port=4
  wires:
  v_actual [m/s]/1 -> Check_Initial_Velocity/1(" v_actual_[m|s]"), Memory External IC/1(u)
  Memory External IC/1(y) -> Sum4/2
  Sum4/1 -> If Desired Velocity ~= 0/2(Desired Velocity [m/s])
  Desired Velocity [m/s]/1 -> if/1, Sum4/1
  Initial Velocity [m/s]/1 -> Check_Initial_Velocity/2(Initial_Velocity_[m|s]), Memory External IC/2(IC), v0 [m/s]/1
  GearNormal/1 -> If Desired Velocity = 0/1(In1)
  Merge/1 -> Demux/1
  If Desired Velocity = 0/1(throttle [%]) -> Mux/1
  If Desired Velocity = 0/2(brake pressure [bar]) -> Mux/2
  Mux2/1 -> Merge/2
  Mux/1 -> Merge/1
  Demux/1 -> throttle [%]/1
  Demux/2 -> brake pressure [bar]/1
  Demux/3 -> Auto_GearShift/1
  "GearNormal "/1 -> If Desired Velocity ~= 0/1(In1)
  If Desired Velocity = 0/3(Auto_GearShift) -> Mux/3
  if/2 -> If Desired Velocity ~= 0/Action
  if/1 -> If Desired Velocity = 0/Action
  If Desired Velocity ~= 0/1(throttle [%]) -> Mux2/1
  If Desired Velocity ~= 0/2(brake pressure [bar]) -> Mux2/2
  If Desired Velocity ~= 0/3(Auto_GearShift) -> Mux2/3

== system ADAC_AEBS_Test_B5_cs/Audi_A8_1/SELF_Demux/compas converter ==
  rotz [rad] : Inport
  cart2compas : Subsystem
  rad2deg : Gain  Gain=180/pi
  heading [deg] : Outport
  wires:
  rad2deg/1 -> cart2compas/1(Angle [deg])
  rotz [rad]/1 -> rad2deg/1
  cart2compas/1(heading [deg]) -> heading [deg]/1

== system ADAC_AEBS_Test_B5_cs/Audi_A8_1/WheelDisplacement_Mux/WheelL0_Mux ==
  X [m] : Inport
  Y [m] : Inport  Port=2
  Z [m] : Inport  Port=3
  Roll [rad] : Inport  Port=4
  Pitch [rad] : Inport  Port=5
  Yaw [rad] : Inport  Port=6
  Bus Creator : BusCreator  Inputs=3  OutDataTypeStr=Bus: PRESCAN_XYZ_DATA
  Bus Creator1 : BusCreator  Inputs=3  OutDataTypeStr=Bus: PRESCAN_RPY_DATA
  Bus Creator2 : BusCreator  Inputs=2  OutDataTypeStr=Bus: PRESCAN_POSE_DATA
  Joint : Outport
  wires:
  Yaw [rad]/1 -> Bus Creator1/3  "Yaw"
  Bus Creator1/1 -> Bus Creator2/2  "ORIENTATION"
  Bus Creator/1 -> Bus Creator2/1  "POSITION"
  X [m]/1 -> Bus Creator/1  "X"
  Y [m]/1 -> Bus Creator/2  "Y"
  Z [m]/1 -> Bus Creator/3  "Z"
  Bus Creator2/1 -> Joint/1
  Roll [rad]/1 -> Bus Creator1/1  "Roll"
  Pitch [rad]/1 -> Bus Creator1/2  "Pitch"

== system ADAC_AEBS_Test_B5_cs/Audi_A8_1/WheelDisplacement_Mux/WheelL1_Mux ==
  X [m] : Inport
  Y [m] : Inport  Port=2
  Z [m] : Inport  Port=3
  Roll [rad] : Inport  Port=4
  Pitch [rad] : Inport  Port=5
  Yaw [rad] : Inport  Port=6
  Bus Creator : BusCreator  Inputs=3  OutDataTypeStr=Bus: PRESCAN_XYZ_DATA
  Bus Creator1 : BusCreator  Inputs=3  OutDataTypeStr=Bus: PRESCAN_RPY_DATA
  Bus Creator2 : BusCreator  Inputs=2  OutDataTypeStr=Bus: PRESCAN_POSE_DATA
  Joint : Outport
  wires:
  Yaw [rad]/1 -> Bus Creator1/3  "Yaw"
  Bus Creator1/1 -> Bus Creator2/2  "ORIENTATION"
  Bus Creator/1 -> Bus Creator2/1  "POSITION"
  X [m]/1 -> Bus Creator/1  "X"
  Y [m]/1 -> Bus Creator/2  "Y"
  Z [m]/1 -> Bus Creator/3  "Z"
  Bus Creator2/1 -> Joint/1
  Roll [rad]/1 -> Bus Creator1/1  "Roll"
  Pitch [rad]/1 -> Bus Creator1/2  "Pitch"

== system ADAC_AEBS_Test_B5_cs/Audi_A8_1/WheelDisplacement_Mux/WheelR0_Mux ==
  X [m] : Inport
  Y [m] : Inport  Port=2
  Z [m] : Inport  Port=3
  Roll [rad] : Inport  Port=4
  Pitch [rad] : Inport  Port=5
  Yaw [rad] : Inport  Port=6
  Bus Creator : BusCreator  Inputs=3  OutDataTypeStr=Bus: PRESCAN_XYZ_DATA
  Bus Creator1 : BusCreator  Inputs=3  OutDataTypeStr=Bus: PRESCAN_RPY_DATA
  Bus Creator2 : BusCreator  Inputs=2  OutDataTypeStr=Bus: PRESCAN_POSE_DATA
  Joint : Outport
  wires:
  Yaw [rad]/1 -> Bus Creator1/3  "Yaw"
  Bus Creator1/1 -> Bus Creator2/2  "ORIENTATION"
  Bus Creator/1 -> Bus Creator2/1  "POSITION"
  X [m]/1 -> Bus Creator/1  "X"
  Y [m]/1 -> Bus Creator/2  "Y"
  Z [m]/1 -> Bus Creator/3  "Z"
  Bus Creator2/1 -> Joint/1
  Roll [rad]/1 -> Bus Creator1/1  "Roll"
  Pitch [rad]/1 -> Bus Creator1/2  "Pitch"

== system ADAC_AEBS_Test_B5_cs/Audi_A8_1/WheelDisplacement_Mux/WheelR1_Mux ==
  X [m] : Inport
  Y [m] : Inport  Port=2
  Z [m] : Inport  Port=3
  Roll [rad] : Inport  Port=4
  Pitch [rad] : Inport  Port=5
  Yaw [rad] : Inport  Port=6
  Bus Creator : BusCreator  Inputs=3  OutDataTypeStr=Bus: PRESCAN_XYZ_DATA
  Bus Creator1 : BusCreator  Inputs=3  OutDataTypeStr=Bus: PRESCAN_RPY_DATA
  Bus Creator2 : BusCreator  Inputs=2  OutDataTypeStr=Bus: PRESCAN_POSE_DATA
  Joint : Outport
  wires:
  Yaw [rad]/1 -> Bus Creator1/3  "Yaw"
  Bus Creator1/1 -> Bus Creator2/2  "ORIENTATION"
  Bus Creator/1 -> Bus Creator2/1  "POSITION"
  X [m]/1 -> Bus Creator/1  "X"
  Y [m]/1 -> Bus Creator/2  "Y"
  Z [m]/1 -> Bus Creator/3  "Z"
  Bus Creator2/1 -> Joint/1
  Roll [rad]/1 -> Bus Creator1/1  "Roll"
  Pitch [rad]/1 -> Bus Creator1/2  "Pitch"

== system ADAC_AEBS_Test_B5_cs/Sphere_1/Dynamics_Empty/MuxState ==
  note: mode: Dynamics
  note: mode: Positioning
  note: mode: Dynamics
      | VelVEHICLE
      | wrt VEH
  note: AnglesVEHICLE
      | wrtGLOB
  note: For state mode 'Dynamic' positions
      | are not taken into account, as they
      | are computed by integrating velocity.
      | Click annotation for Help.
  x [m] : Inport  SampleTime=TimeStep
  y [m] : Inport  Port=2  SampleTime=TimeStep
  z [m] : Inport  Port=3  SampleTime=TimeStep
  dx [m/s] : Inport  Port=4  SampleTime=TimeStep
  dy [m/s] : Inport  Port=5  SampleTime=TimeStep
  dz [m/s] : Inport  Port=6  SampleTime=TimeStep
  R [rad] : Inport  Port=7  SampleTime=TimeStep
  P [rad] : Inport  Port=8  SampleTime=TimeStep
  Y [rad] : Inport  Port=9  SampleTime=TimeStep
  Constant : Constant  DisableCoverage=on  Value=positioningmode
  Discrete-Time Integrator : DiscreteIntegrator  SampleTime=TimeStep
  Ground : Ground
  Ground1 : Ground
  Mux1 : Mux  Inputs=[3 3]
  Mux2 : Mux  Inputs=3
  Mux3 : Mux  Inputs=3
  Mux4 : Mux  Inputs=3
  Mux5 : Mux  Inputs=[3 3]
  Mux6 : Mux  Inputs=[6 3]
  Switch : Switch  Threshold=0.5
  Transformation_BODY2GLOBAL : PreScanSimulinkLibrary/Simple_Vehicle_Dynamics/Chassis/MuxDynState/Transformation_BODY2GLOBAL
  mux3 : Mux  Inputs=3
  state : Outport
  wires:
  Constant/1 -> Switch/2
  Mux6/1 -> state/1
  Mux4/1 -> Mux1/1
  Mux5/1 -> Switch/3
  Mux1/1 -> Switch/1
  Switch/1 -> Mux6/1  "PosVeh wrt  GLOB"
  P [rad]/1 -> Mux3/2
  R [rad]/1 -> Mux3/1
  dz [m/s]/1 -> Mux2/3
  dy [m/s]/1 -> Mux2/2
  dx [m/s]/1 -> Mux2/1
  z [m]/1 -> Mux4/3
  y [m]/1 -> Mux4/2
  x [m]/1 -> Mux4/1
  Ground1/1 -> mux3/2  "pitch"
  Y [rad]/1 -> mux3/3, Mux3/3  "yaw"
  Mux3/1 -> Mux6/2
  Transformation_BODY2GLOBAL/1 -> Discrete-Time Integrator/1, Mux5/2  "VelVEH wrt  GLOB"
  mux3/1 -> Transformation_BODY2GLOBAL/2
  Ground/1 -> mux3/1  "roll"
  Mux2/1 -> Mux1/2, Transformation_BODY2GLOBAL/1
  Discrete-Time Integrator/1 -> Mux5/1  "PosVEH wrt  GLOB"

== system ADAC_AEBS_Test_B5_cs/Sphere_1/Dynamics_Empty/STATE_Sphere_1 ==
  State : Inport  SampleTime=TimeStep
  Bus Creator : BusCreator  Inputs=15  OutDataTypeStr=Bus: PRESCAN_STATEACTUATORDATA  NonVirtualBus=on
  Constant : Constant  Value=0
  Demux : Demux  Outputs=15
  Mux : Mux  Inputs=3
  Mux1 : Mux  Inputs=3
  Mux2 : Mux  Inputs=3
  iniBODYAngles wrtVEH [rad] : Constant  Value=Roll0  SampleTime=TimeStep
  iniBODYAngles wrtVEH [rad]1 : Constant  Value=Pitch0  SampleTime=TimeStep
  iniVEHAngles wrtGLOB [rad] : Constant  Value=Yaw0  SampleTime=TimeStep
  iniVEHposition wrtGLOB [m] : Constant  Value=x0  SampleTime=TimeStep
  iniVEHposition wrtGLOB [m]1 : Constant  Value=y0  SampleTime=TimeStep
  iniVEHposition wrtGLOB [m]2 : Constant  Value=z0  SampleTime=TimeStep
  state2FullState : PreScanSimulinkLibrary/state2FullState  SystemSampleTime=-1
  StateBus : Outport  OutDataTypeStr=Bus: PRESCAN_STATEACTUATORDATA
  wires:
  Mux2/1 -> state2FullState/4
  iniVEHAngles wrtGLOB [rad]/1 -> Mux2/3
  Mux1/1 -> state2FullState/3
  Constant/1 -> Mux2/1, Mux2/2, Mux1/3
  iniBODYAngles wrtVEH [rad]1/1 -> Mux1/2
  iniBODYAngles wrtVEH [rad]/1 -> Mux1/1
  Mux/1 -> state2FullState/2
  iniVEHposition wrtGLOB [m]2/1 -> Mux/3
  iniVEHposition wrtGLOB [m]/1 -> Mux/1
  iniVEHposition wrtGLOB [m]1/1 -> Mux/2
  Demux/15 -> Bus Creator/15  "AngularVelocityYaw"
  Demux/14 -> Bus Creator/14  "AngularVelocityPitch"
  Demux/13 -> Bus Creator/13  "AngularVelocityRoll"
  Demux/12 -> Bus Creator/12  "OrientationYaw"
  Demux/11 -> Bus Creator/11  "OrientationPitch"
  Demux/10 -> Bus Creator/10  "OrientationRoll"
  Demux/9 -> Bus Creator/9  "AccelerationZ"
  Demux/8 -> Bus Creator/8  "AccelerationY"
  Demux/7 -> Bus Creator/7  "AccelerationX"
  Demux/6 -> Bus Creator/6  "VelocityZ"
  Demux/5 -> Bus Creator/5  "VelocityY"
  Demux/4 -> Bus Creator/4  "VelocityX"
  Demux/3 -> Bus Creator/3  "PositionZ"
  Demux/2 -> Bus Creator/2  "PositionY"
  Demux/1 -> Bus Creator/1  "PositionX"
  state2FullState/1 -> Demux/1
  State/1 -> state2FullState/1
  Bus Creator/1 -> StateBus/1

== system ADAC_AEBS_Test_B5_cs/Sphere_1/SELF_Demux/compas converter ==
  rotz [rad] : Inport
  cart2compas : Subsystem
  rad2deg : Gain  Gain=180/pi
  heading [deg] : Outport
  wires:
  rad2deg/1 -> cart2compas/1(Angle [deg])
  rotz [rad]/1 -> rad2deg/1
  cart2compas/1(heading [deg]) -> heading [deg]/1

== system ADAC_AEBS_Test_B5_cs/SteeringColumn_pivot_Audi_A8_1/Actuator/visu_Rotate ==
  In1 : Inport
  sfun_RPYActuator : S-Function  FunctionName=sfun_RPYActuator  Parameters=SParameter1, SParameter2, SampleTime  EnableBusSupport=off  mask(Legacy Function){SFunctionSpec=void prescan_outputFcn(void ** work1,  PRESCAN_XYZ_DATA u1[1]), SParameter1=UniqueID, SParameter2=uint8([Object3DID 0]), SampleTime=TimeStep, ShowSpec=on}
      mask prompts: SParameter1 "P1:"; SParameter2 "P2:"; SampleTime "Sample time (-1 for inherited):"; ShowSpec "Display function specification"
      mask help:
      | This block allows you to call the legacy functions specified by the following Legacy Code Tool definition:
      | def.SFunctionName = 'sfun_PositionActuator';
      | def.OutputFcnSpec = 'void prescan_outputFcn(void ** work1,  PRESCAN_XYZ_DATA u1[1])';
      | def.StartFcnSpec = 'void prescan_startFcn(void ** work1, uint8 p1[], double p2)';
      | def.TerminateFcnSpec = 'void prescan_terminateFcn(void ** work1)';
      | def.HeaderFiles = {'prescan_positionactuator_data.h', 'prescan_header_data.h', 'prescan_SFunLibrary.h', 'prescan_CreateLogHandler.h', 'prescan_CreateErrorHandler.h'};
      | def.SourceFiles = {'prescan_MexLogHandler.cpp', 'prescan_SimStructErrorHandler.cpp', 'prescan_ConcurrentLogHandler.cpp', 'prescan_ConcurrentErrorHandler.cpp'};
      | def.HostLibFiles = {'sensorinterfaced.lib'};
      | def.TargetLibFiles = {'sensorinterfaced.so'};
      | def.IncPaths = {'.', 'C:\prescandev\vislibrary\vis\..\pimp\include\sensors\InterfaceRTW'};
      | def.SrcPaths = {'.'};
      | def.LibPaths = {'C:\\prescandev\\vislibrary_build\lib'};
      | def.SampleTime = 'parameterized';
      mask Help: <p>This block was generated automatically by the Legacy Code Tool. For detailed help on this tool, call<a href="matlab:legacy_code('help')"> legacy_code('help')</a>.</p>
      mask Callback ShowSpec:
      | if strcmp(get_param(gcbh, 'ShowSpec'), 'on')
      |   set_param(gcbh, 'MaskDisplay', sprintf('fprintf(''%s'');', get_param(gcbh, 'SFunctionSpec')));
      | else
      |   set_param(gcbh, 'MaskDisplay', sprintf('fprintf(''%s'');', get_param(gcbh, 'FunctionName')));
      | end
      mask Display: fprintf('void prescan_outputFcn(void ** work1,  PRESCAN_RPY_DATA u1[1])');
  wires:
  In1/1 -> sfun_RPYActuator/1

== system ADAC_AEBS_Test_B5_cs/SteeringColumn_pivot_Audi_A8_1/Actuator/visu_Translate ==
  In1 : Inport
  sfun_PositionActuator : S-Function  FunctionName=sfun_PositionActuator  Parameters=SParameter1, SParameter2, SampleTime  EnableBusSupport=off  mask(Legacy Function){SFunctionSpec=void prescan_outputFcn(void ** work1,  PRESCAN_XYZ_DATA u1[1]), SParameter1=uint8([Object3DID 0]), SParameter2=UniqueID, SampleTime=TimeStep, ShowSpec=on}
      mask prompts: SParameter1 "P1:"; SParameter2 "P2:"; SampleTime "Sample time (-1 for inherited):"; ShowSpec "Display function specification"
      mask help:
      | This block allows you to call the legacy functions specified by the following Legacy Code Tool definition:
      | def.SFunctionName = 'sfun_PositionActuator';
      | def.OutputFcnSpec = 'void prescan_outputFcn(void ** work1,  PRESCAN_XYZ_DATA u1[1])';
      | def.StartFcnSpec = 'void prescan_startFcn(void ** work1, uint8 p1[], double p2)';
      | def.TerminateFcnSpec = 'void prescan_terminateFcn(void ** work1)';
      | def.HeaderFiles = {'prescan_positionactuator_data.h', 'prescan_header_data.h', 'prescan_SFunLibrary.h', 'prescan_CreateLogHandler.h', 'prescan_CreateErrorHandler.h'};
      | def.SourceFiles = {'prescan_MexLogHandler.cpp', 'prescan_SimStructErrorHandler.cpp', 'prescan_ConcurrentLogHandler.cpp', 'prescan_ConcurrentErrorHandler.cpp'};
      | def.HostLibFiles = {'sensorinterfaced.lib'};
      | def.TargetLibFiles = {'sensorinterfaced.so'};
      | def.IncPaths = {'.', 'C:\prescandev\vislibrary\vis\..\pimp\include\sensors\InterfaceRTW'};
      | def.SrcPaths = {'.'};
      | def.LibPaths = {'C:\\prescandev\\vislibrary_build\lib'};
      | def.SampleTime = 'parameterized';
      mask Help: <p>This block was generated automatically by the Legacy Code Tool. For detailed help on this tool, call<a href="matlab:legacy_code('help')"> legacy_code('help')</a>.</p>
      mask Callback ShowSpec:
      | if strcmp(get_param(gcbh, 'ShowSpec'), 'on')
      |   set_param(gcbh, 'MaskDisplay', sprintf('fprintf(''%s'');', get_param(gcbh, 'SFunctionSpec')));
      | else
      |   set_param(gcbh, 'MaskDisplay', sprintf('fprintf(''%s'');', get_param(gcbh, 'FunctionName')));
      | end
      mask Display: fprintf('void prescan_outputFcn(void ** work1,  PRESCAN_XYZ_DATA u1[1])');
  wires:
  In1/1 -> sfun_PositionActuator/1

== system ADAC_AEBS_Test_B5_cs/SteeringWheel_pivot_Audi_A8_1/Actuator/visu_Rotate ==
  In1 : Inport
  sfun_RPYActuator : S-Function  FunctionName=sfun_RPYActuator  Parameters=SParameter1, SParameter2, SampleTime  EnableBusSupport=off  mask(Legacy Function){SFunctionSpec=void prescan_outputFcn(void ** work1,  PRESCAN_XYZ_DATA u1[1]), SParameter1=UniqueID, SParameter2=uint8([Object3DID 0]), SampleTime=TimeStep, ShowSpec=on}
      mask prompts: SParameter1 "P1:"; SParameter2 "P2:"; SampleTime "Sample time (-1 for inherited):"; ShowSpec "Display function specification"
      mask help:
      | This block allows you to call the legacy functions specified by the following Legacy Code Tool definition:
      | def.SFunctionName = 'sfun_PositionActuator';
      | def.OutputFcnSpec = 'void prescan_outputFcn(void ** work1,  PRESCAN_XYZ_DATA u1[1])';
      | def.StartFcnSpec = 'void prescan_startFcn(void ** work1, uint8 p1[], double p2)';
      | def.TerminateFcnSpec = 'void prescan_terminateFcn(void ** work1)';
      | def.HeaderFiles = {'prescan_positionactuator_data.h', 'prescan_header_data.h', 'prescan_SFunLibrary.h', 'prescan_CreateLogHandler.h', 'prescan_CreateErrorHandler.h'};
      | def.SourceFiles = {'prescan_MexLogHandler.cpp', 'prescan_SimStructErrorHandler.cpp', 'prescan_ConcurrentLogHandler.cpp', 'prescan_ConcurrentErrorHandler.cpp'};
      | def.HostLibFiles = {'sensorinterfaced.lib'};
      | def.TargetLibFiles = {'sensorinterfaced.so'};
      | def.IncPaths = {'.', 'C:\prescandev\vislibrary\vis\..\pimp\include\sensors\InterfaceRTW'};
      | def.SrcPaths = {'.'};
      | def.LibPaths = {'C:\\prescandev\\vislibrary_build\lib'};
      | def.SampleTime = 'parameterized';
      mask Help: <p>This block was generated automatically by the Legacy Code Tool. For detailed help on this tool, call<a href="matlab:legacy_code('help')"> legacy_code('help')</a>.</p>
      mask Callback ShowSpec:
      | if strcmp(get_param(gcbh, 'ShowSpec'), 'on')
      |   set_param(gcbh, 'MaskDisplay', sprintf('fprintf(''%s'');', get_param(gcbh, 'SFunctionSpec')));
      | else
      |   set_param(gcbh, 'MaskDisplay', sprintf('fprintf(''%s'');', get_param(gcbh, 'FunctionName')));
      | end
      mask Display: fprintf('void prescan_outputFcn(void ** work1,  PRESCAN_RPY_DATA u1[1])');
  wires:
  In1/1 -> sfun_RPYActuator/1
